simulink library "planarBAT_ul"  (R2018b)
settings: Solver=VariableStepAuto  StartTime=0.0  StopTime=10.0  RelTol=1e-3
libraries: vrlib x1
settings Model: Creator=Ayaz  LastModifiedBy=Ayaz

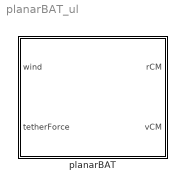
== system planarBAT_ul ==
  planarBAT : Subsystem  mask{rhoF=1, gravAcc=9.81, mT=1, BF=1.5, Sref=1, Cd=0.5, ini_rCM=[0; 100], ini_vCM=[0;0]}
      mask prompts: rhoF "Fluid density"; gravAcc "Gravitational acceleration"; mT "Mass"; BF "Buoyancy factor"; Sref "Reference area"; Cd "Drag coefficient"; ini_rCM "Initial position"; ini_vCM "Initial velocity"
      mask init:
      | F_grav = mT*gravAcc*[0;-1];
      | F_buoy = -F_grav.*BF;
      mask DialogControl ParameterGroupVar Prompt: Environment
      mask DialogControl Container3 Prompt: Body
      mask DialogControl Container4 Prompt: Initial condition

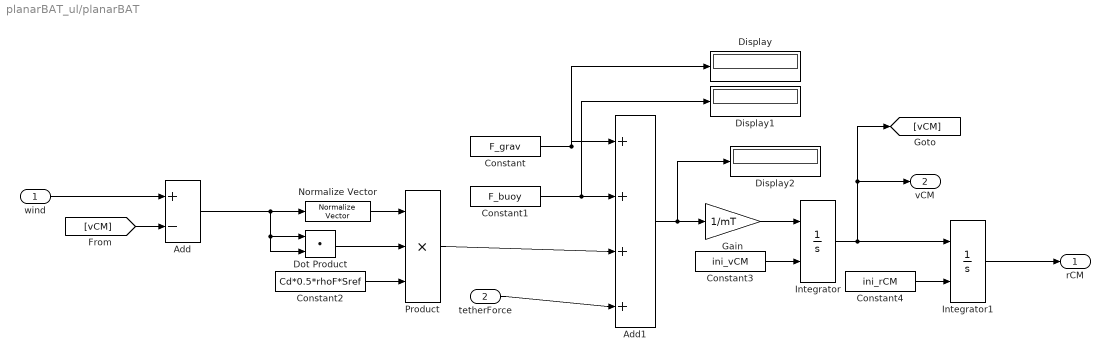
== system planarBAT_ul/planarBAT ==
  wind : Inport
  tetherForce : Inport  Port=2
  Add : Sum  Inputs=+-
  Add1 : Sum  Inputs=++++
  Constant : Constant  Value=F_grav  VectorParams1D=off
  Constant1 : Constant  Value=F_buoy  VectorParams1D=off
  Constant2 : Constant  Value=Cd*0.5*rhoF*Sref  VectorParams1D=off
  Constant3 : Constant  Value=ini_vCM  VectorParams1D=off
  Constant4 : Constant  Value=ini_rCM  VectorParams1D=off
  Display : Display
  Display1 : Display
  Display2 : Display
  Dot Product : DotProduct  InputSameDT=on  OutDataTypeStr=Inherit: Inherit via internal rule
  Gain : Gain  Gain=1/mT
  Integrator : Integrator  InitialConditionSource=external
  Integrator1 : Integrator  InitialConditionSource=external
  Normalize Vector : vrlib/Utilities/Normalize Vector  maxzero=0
      settings: SourceProductName=Simulink 3D Animation  SourceProductBaseCode=VR
  Product : Product  Inputs=3
  rCM : Outport
  vCM : Outport  Port=2
  wires:
  wind/1 -> Add/1
  [vCM] -> Add/2
  Add/1 -> Dot Product/2, Dot Product/1, Normalize Vector/1
  Normalize Vector/1 -> Product/1
  Dot Product/1 -> Product/2
  Constant2/1 -> Product/3
  Product/1 -> Add1/3
  tetherForce/1 -> Add1/4
  Constant1/1 -> Display1/1, Add1/2
  Constant/1 -> Display/1, Add1/1
  Add1/1 -> Display2/1, Gain/1
  Gain/1 -> Integrator/1
  Constant3/1 -> Integrator/2
  Integrator/1 -> [vCM], vCM/1, Integrator1/1
  Constant4/1 -> Integrator1/2
  Integrator1/1 -> rCM/1
